simulink model "water_tank"  (R2024b)
settings: Solver=VariableStepAuto  StartTime=0.0  StopTime=10.0  RelTol=1e-3

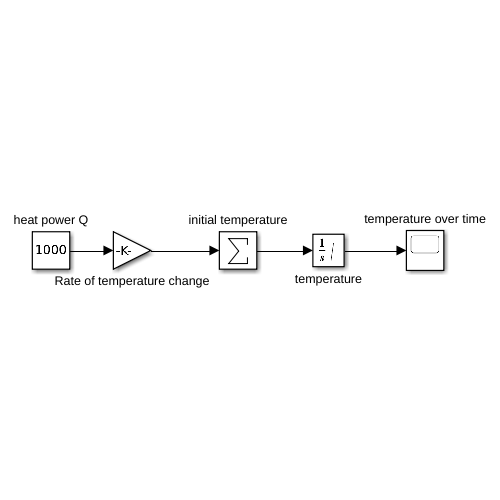
[thumbnail: Simulink's stored preview of the top-level diagram]
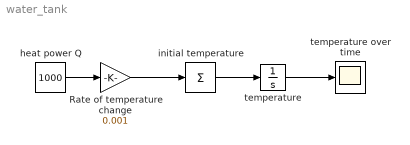
== system water_tank ==
  Rate of temperature change : Gain  Gain=0.001
  heat power Q : Constant  Value=1000
  initial temperature : Sum  Inputs=+
  temperature : Integrator  InitialCondition=20  LimitOutput=on  UpperSaturationLimit=100  LowerSaturationLimit=0
  temperature over time : Scope
  wires:
  heat power Q/1 -> Rate of temperature change/1
  Rate of temperature change/1 -> initial temperature/1
  initial temperature/1 -> temperature/1
  temperature/1 -> temperature over time/1
